simulink model "VehCtrlMdel240926_2018b"  (R2019b)
settings: Solver=FixedStepDiscrete  StartTime=0.0  StopTime=10.0  FixedStep=0.0005  RelTol=1e-3  EnableMultiTasking=on
values from neighbouring files (symbols this model uses):
  Ax_OffSet = 0.0    [VehCtrlMdelDictionary.sldd]
  Ay_OffSet = 0.0    [VehCtrlMdelDictionary.sldd]
  Caf = 460.0    [VehCtrlMdelDictionary.sldd]    (also in trqvparameter.m = 460)
  Car = 440.0    [VehCtrlMdelDictionary.sldd]    (also in trqvparameter.m = 440)
  dwf = 1.2    [VehCtrlMdelDictionary.sldd]    (also in trqvparameter.m)
  dwr = 1.2    [VehCtrlMdelDictionary.sldd]    (also in trqvparameter.m)
  h = 0.29    [VehCtrlMdelDictionary.sldd]    (also in trqvparameter.m)
  i1 = 11.4    [VehCtrlMdelDictionary.sldd]    (also in trqvparameter.m)
  i2 = 3.4    [VehCtrlMdelDictionary.sldd]    (also in trqvparameter.m)
  Iz = 105.0    [VehCtrlMdelDictionary.sldd]    (also in trqvparameter.m = 105)
  Kc = 1.0    [VehCtrlMdelDictionary.sldd]    (also in trqvparameter.m = 10)
  Ki = 1.0    [VehCtrlMdelDictionary.sldd]    (also in trqvparameter.m = 20)
  Kp = 2.0    [VehCtrlMdelDictionary.sldd]    (also in trqvparameter.m = 30)
  Ldwf = 1.2    [VehCtrlMdelDictionary.sldd]    (also in trqvparameter.m)
  Ldwr = 1.16    [VehCtrlMdelDictionary.sldd]    (also in trqvparameter.m)
  lf = 0.761    [VehCtrlMdelDictionary.sldd]    (also in trqvparameter.m)
  lr = 0.831    [VehCtrlMdelDictionary.sldd]    (also in trqvparameter.m)
  m = 340.0    [VehCtrlMdelDictionary.sldd]    (also in trqvparameter.m = 340)
  Offset_Angle = 0.0    [VehCtrlMdelDictionary.sldd]
  Qa = 0.1    [VehCtrlMdelDictionary.sldd]    (also in trqvparameter.m)
  Ra = 2.0    [VehCtrlMdelDictionary.sldd]    (also in trqvparameter.m = 2)
  Rt = 0.2    [VehCtrlMdelDictionary.sldd]    (also in trqvparameter.m)
  thr1 = 2.0    [VehCtrlMdelDictionary.sldd]    (also in trqvparameter.m = 2)
  thr2 = 0.5    [VehCtrlMdelDictionary.sldd]    (also in trqvparameter.m)
  thr3 = 0.8    [VehCtrlMdelDictionary.sldd]    (also in trqvparameter.m)
  thr4 = 0.5    [VehCtrlMdelDictionary.sldd]    (also in trqvparameter.m)
  thr5 = -0.5    [VehCtrlMdelDictionary.sldd]    (also in trqvparameter.m)
  TrqRquRate = 0.1    [VehCtrlMdelDictionary.sldd]    (also in trqvparameter.m)
  YawRate_OffSet = 0.0    [VehCtrlMdelDictionary.sldd]
undefined symbols (not defined in the file or in its folder): DiscIntNeverNeededParam, I_AN06_5V, I_AN07_5V, I_AN08_5V, I_AN09_5V, I_SW01_L, I_SW03_L, O_SW12_HS1A, O_SW14_HS1A, PWM3
libraries: simulink x150, ec5744lib x118, canmsglib x18
(part 2 of 6)

== system VehCtrlMdel240926_2018b/OUTPUT/VCU2AMKMCUFL ==
  MCFL_TargetTorque : Inport
  In2 : Inport  Port=2
  function : TriggerPort  TriggerType=function-call  VariantControl=(inherit)
  Bus Selector : BusSelector  OutputSignals=MCFL_TorqueOn,MCFL_DCOn_setpoints,MCFL_DCEnable,errorReset,MCFL_InverterOn
  CAN Pack1 : canmsglib/CAN Pack  CANdbFile=C:\Users\12045\Desktop\DBC\DRe20_dbc_v1.16\DRe20_dbc_v1.16_CAN2.dbc  MsgList=MCFL_SetPoints  MsgName=MCFL_SetPoints  MsgIDType=Standard (11-bit identifier)  MsgIdentifier=386  MsgLength=8  Remote=off  ApplyMinMax=off  BusOutput=off  SignalInfo={'MCFL_TargetTorque','16','16','LE','signed','Standard','0','0.0098','0','-Inf','Inf';'MCFL_TorqueLimitN','48','16','LE','signed','Standard','0','0.0098','0','-Inf','Inf';'MCFL_TorqueLimitP','32','16','LE','signed','Standard','0','0.0098','0','-Inf','Inf';'MCFL_cDCOn','9','1','LE','unsigned','Standard','0','1','0','0','1';'MCFL_cEnable','10','1','LE','unsigned','Standard','0','1','0','0','1';'MCFL_cErrorReset','11','1','LE','unsigned','Standard','0','1','0','0','1';'MCFL_cInverterOn','8','1','LE','unsigned','Standard','0','1','0','0','1';'MCFL_cReserve1','0','8','LE','unsigned','Standard','0','1','0','-Inf','Inf';'MCFL_cReserve2','12','4','LE','unsigned','Standard','0','1','0','-Inf','Inf'}
      settings: SourceProductName=Vehicle Network Toolbox  SourceProductBaseCode=VN  DataFormat=CANdb specified signals
  CANPackMessage : ec5744lib/RapidECU_U3/04CANCommunication/CANPackMessage  datalength=8  sampletime=-1
      settings: SourceProductName=ECUCoder for MPC5744
  CANTransmit : ec5744lib/RapidECU_U3/04CANCommunication/CANTransmit  canmodule=1  canbuffer=8  canmessageid=386  canmessagetype=Standard(11-bit ID)  datalength=8  sampletime=-1
      settings: SourceProductName=ECUCoder for MPC5744
  Constant1 : Constant  Value=0
  Constant2 : Constant  Value=10
  Ground1 : Ground
  Ground2 : Ground
  Switch : Switch  Criteria=u2 ~= 0
  Terminator3 : Terminator
  wires:
  CANPackMessage/1 -> CANTransmit/1
  CAN Pack1/1 -> CANPackMessage/1
  CANTransmit/1 -> Terminator3/1
  MCFL_TargetTorque/1 -> CAN Pack1/1  "MCFL_TargetTorque"
  Constant1/1 -> CAN Pack1/2, Switch/3  "MCFL_TorqueLimitN"
  Bus Selector/2 -> CAN Pack1/4  "<MCFL_DCOn_setpoints>"
  Switch/1 -> CAN Pack1/3  "MCFL_TorqueLimitP"
  Ground1/1 -> CAN Pack1/8  "MCFL_cReserve1"
  Bus Selector/5 -> CAN Pack1/7  "<MCFL_InverterOn>"
  Bus Selector/3 -> CAN Pack1/5  "<MCFL_DCEnable>"
  Ground2/1 -> CAN Pack1/9  "MCFL_cReserve2"
  In2/1 -> Bus Selector/1
  Bus Selector/4 -> CAN Pack1/6  "<errorReset>"
  Bus Selector/1 -> Switch/2  "<MCFL_TorqueOn>"
  Constant2/1 -> Switch/1  "MCFL_TorqueLimitP"

== system VehCtrlMdel240926_2018b/OUTPUT/VCU2AMKMCUFR ==
  <BUS> : Inport
  In1 : Inport  Port=2
  function : TriggerPort  TriggerType=function-call  VariantControl=(inherit)
  Bus Selector : BusSelector  OutputSignals=MCFR_TorqueOn,MCFL_DCOn_setpoints,MCFL_DCEnable,errorReset,MCFL_InverterOn
  CAN Pack1 : canmsglib/CAN Pack  CANdbFile=C:\Users\12045\Desktop\DBC\DRe20_dbc_v1.16\DRe20_dbc_v1.16_CAN2.dbc  MsgList=MCFR_SetPoints  MsgName=MCFR_SetPoints  MsgIDType=Standard (11-bit identifier)  MsgIdentifier=387  MsgLength=8  Remote=off  ApplyMinMax=off  BusOutput=off  SignalInfo={'MCFR_TargetTorque','16','16','LE','signed','Standard','0','0.0098','0','-Inf','Inf';'MCFR_TorqueLimitN','48','16','LE','signed','Standard','0','0.0098','0','-Inf','Inf';'MCFR_TorqueLimitP','32','16','LE','signed','Standard','0','0.0098','0','-Inf','Inf';'MCFR_cDCOn','9','1','LE','unsigned','Standard','0','1','0','0','1';'MCFR_cEnable','10','1','LE','unsigned','Standard','0','1','0','0','1';'MCFR_cErrorReset','11','1','LE','unsigned','Standard','0','1','0','0','1';'MCFR_cInverterOn','8','1','LE','unsigned','Standard','0','1','0','0','1';'MCFR_cReserve1','0','8','LE','unsigned','Standard','0','1','0','-Inf','Inf';'MCFR_cReserve2','12','4','LE','unsigned','Standard','0','1','0','-Inf','Inf'}
      settings: SourceProductName=Vehicle Network Toolbox  SourceProductBaseCode=VN  DataFormat=CANdb specified signals
  CANPackMessage : ec5744lib/RapidECU_U3/04CANCommunication/CANPackMessage  datalength=8  sampletime=-1
      settings: SourceProductName=ECUCoder for MPC5744
  CANTransmit : ec5744lib/RapidECU_U3/04CANCommunication/CANTransmit  canmodule=1  canbuffer=9  canmessageid=387  canmessagetype=Standard(11-bit ID)  datalength=8  sampletime=-1
      settings: SourceProductName=ECUCoder for MPC5744
  Constant : Constant  Value=0
  Constant1 : Constant  Value=10
  Ground : Ground
  Ground1 : Ground
  Switch : Switch  Criteria=u2 ~= 0
  Terminator3 : Terminator
  wires:
  Ground1/1 -> CAN Pack1/9  "MCFR_cReserve2"
  Bus Selector/3 -> CAN Pack1/5  "<MCFL_DCEnable>"
  Bus Selector/4 -> CAN Pack1/6  "<errorReset>"
  Bus Selector/5 -> CAN Pack1/7  "<MCFL_InverterOn>"
  Ground/1 -> CAN Pack1/8  "MCFR_cReserve1"
  Switch/1 -> CAN Pack1/3  "MCFR_TorqueLimitP"
  Bus Selector/2 -> CAN Pack1/4  "<MCFL_DCOn_setpoints>"
  Constant/1 -> CAN Pack1/2, Switch/3  "MCFR_TorqueLimitN"
  CANTransmit/1 -> Terminator3/1
  CAN Pack1/1 -> CANPackMessage/1
  CANPackMessage/1 -> CANTransmit/1
  In1/1 -> CAN Pack1/1
  <BUS>/1 -> Bus Selector/1
  Constant1/1 -> Switch/1  "MCFR_TorqueLimitP"
  Bus Selector/1 -> Switch/2  "<MCFR_TorqueOn>"

== system VehCtrlMdel240926_2018b/OUTPUT/VCU2CLUSTER ==
  In1 : Inport
  TCS : Inport  Port=2
  function : TriggerPort  TriggerType=function-call  VariantControl=Variant
  Bus Selector : BusSelector  OutputSignals=signal2.APPBrk_BUS.Brk_F,signal2.MCU.MCU_state.Trq,signal2.APPBrk_BUS.Acc_POS,signal2.MCU.MCU_pwr.motor_temp,signal2.VehSpd_FLkph,signal2.MCU.MCU_state.Spd_R_kph,signal2.APPBrk_BUS.Brk_R,signal2.MCU.MCU_state.RPM
  Bus Selector1 : BusSelector  OutputSignals=TCS_TrqRequestFinal_Nm,TCS_flgActv
  CAN Pack : canmsglib/CAN Pack  CANdbFile=E:\candbc\cluster.dbc  MsgList=(none)  MsgName=New_Message_1  MsgIDType=Standard (11-bit identifier)  MsgIdentifier=291  MsgLength=8  Remote=off  ApplyMinMax=off  BusOutput=off  SignalInfo={'Brk_F','56','8','LE','signed','Standard','0','30','100','-3740','3910';'TCS_Trq_cmd','40','8','LE','unsigned','Standard','0','1','0','0','255';'TCS_flag','32','8','LE','signed','Standard','0','1','0','-Inf','Inf';'Trq_feedback','48','8','LE','signed','Standard','0','1','0','-128','250';'acc','24','8','LE','unsigned','Standard','0','1','0','0','100';'motor_temp','0','8','LE','unsigned','Standard','0','1','0','0','100';'veh_spd_F','8','8','LE','unsigned','Standard','0','1','0','0','120';'veh_spd_R','16','8','LE','unsigned','Standard','0','1','0','0','120'}
      settings: SourceProductName=Vehicle Network Toolbox  SourceProductBaseCode=VN  DataFormat=CANdb specified signals
  CAN Pack1 : canmsglib/CAN Pack  CANdbFile=E:\candbc\cluster.dbc  MsgList=(none)  MsgName=New_Message_2  MsgIDType=Standard (11-bit identifier)  MsgIdentifier=292  MsgLength=2  Remote=off  ApplyMinMax=off  BusOutput=off  SignalInfo={'Brk_R','0','8','LE','signed','Standard','0','30','100','-Inf','Inf';'RPM_feedback','8','8','LE','signed','Standard','0','1','0','-Inf','Inf'}
      settings: SourceProductName=Simulink Real-Time  SourceProductBaseCode=XP  DataFormat=CANdb specified signals
  CANPackMessage : ec5744lib/RapidECU_U3/04CANCommunication/CANPackMessage  datalength=8  sampletime=-1
      settings: SourceProductName=ECUCoder for MPC5744
  CANPackMessage1 : ec5744lib/HYFCU001/04CANCommunication/CANPackMessage  datalength=8  sampletime=-1
      settings: SourceProductName=ECUCoder for MPC5744
  CANTransmit : ec5744lib/RapidECU_U3/04CANCommunication/CANTransmit  canmodule=0  canbuffer=9  canmessageid=291  canmessagetype=Standard(11-bit ID)  datalength=8  sampletime=-1
      settings: SourceProductName=ECUCoder for MPC5744
  CANTransmit1 : ec5744lib/RapidECU_U3/04CANCommunication/CANTransmit  canmodule=0  canbuffer=10  canmessageid=292  canmessagetype=Standard(11-bit ID)  datalength=8  sampletime=-1
      settings: SourceProductName=ECUCoder for MPC5744
  Terminator1 : Terminator
  Terminator3 : Terminator
  wires:
  CANTransmit/1 -> Terminator3/1
  CANPackMessage/1 -> CANTransmit/1
  CAN Pack/1 -> CANPackMessage/1
  In1/1 -> Bus Selector/1
  Bus Selector/5 -> CAN Pack/7  "<VehSpd_FLkph>"
  Bus Selector/4 -> CAN Pack/6  "<motor_temp>"
  Bus Selector/3 -> CAN Pack/5  "<Acc_POS>"
  Bus Selector/6 -> CAN Pack/8  "<Spd_R_kph>"
  Bus Selector/1 -> CAN Pack/1  "<Brk_F>"
  Bus Selector/2 -> CAN Pack/4  "<Trq>"
  TCS/1 -> Bus Selector1/1
  Bus Selector1/2 -> CAN Pack/3  "<TCS_flgActv>"
  Bus Selector1/1 -> CAN Pack/2  "<TCS_TrqRequestFinal_Nm>"
  Bus Selector/7 -> CAN Pack1/1  "<Brk_R>"
  Bus Selector/8 -> CAN Pack1/2  "<RPM>"
  CAN Pack1/1 -> CANPackMessage1/1
  CANPackMessage1/1 -> CANTransmit1/1
  CANTransmit1/1 -> Terminator1/1

== system VehCtrlMdel240926_2018b/OUTPUT/VCU2EmraxMCU ==
  note: 0: 0Nm
      | 2: Trq mode
  note: 0: N
      | 2:D
  note: 加ramp
  note: 1.spd改成motor_rpm
      | 2.APP_bad改成acc_error
      | 3.设置模式的优先级
      | 4.车轮低负载（悬空），加最高车速限制
  In1 : Inport
  function : TriggerPort  TriggerType=function-call  VariantControl=(inherit)
  Bus Selector : BusSelector  OutputSignals=Trq_CUT,TrqR_cmd,VCU_SpdCmd_Emrax
  CAN Pack1 : canmsglib/CAN Pack  CANdbFile=E:\candbc\MCU_No1.dbc  MsgList=(none)  MsgName=VCU2MCU1_ID1  MsgIDType=Extended (29-bit identifier)  MsgIdentifier=146927393  MsgLength=8  Remote=off  ApplyMinMax=off  BusOutput=off  SignalInfo={'VCU2MCU_Control_mode_ID1','32','8','LE','unsigned','Standard','0','1','0','0','255';'VCU2MCU_Gear_ID1','40','2','LE','unsigned','Standard','0','1','0','0','3';'VCU2MCU_Speed_Limit_ID1','0','16','LE','unsigned','Standard','0','5.000000e-01','-10000','-10000','10000';'VCU2MCU_Torque_Control_ID1','16','16','LE','unsigned','Standard','0','1','0','0','1000'}
      settings: SourceProductName=Vehicle Network Toolbox  SourceProductBaseCode=VN  DataFormat=CANdb specified signals
  CANPackMessage : ec5744lib/RapidECU_U3/04CANCommunication/CANPackMessage  datalength=8  sampletime=-1
      settings: SourceProductName=ECUCoder for MPC5744
  CANTransmit : ec5744lib/RapidECU_U3/04CANCommunication/CANTransmit  canmodule=0  canbuffer=8  canmessageid=146927393  canmessagetype=Extended(29-bit ID)  datalength=8  sampletime=-1
      settings: SourceProductName=ECUCoder for MPC5744
  Cast To Boolean4 : DataTypeConversion  OutDataTypeStr=uint16
  Cast To Boolean6 : DataTypeConversion  OutDataTypeStr=uint16
  Constant13 : Constant  Value=2
  Constant17 : Constant  Value=0
  Constant19 : Constant  Value=2
  Constant20 : Constant  Value=0
  Data Type Conversion1 : DataTypeConversion  OutDataTypeStr=single
  Data Type Conversion2 : DataTypeConversion  OutDataTypeStr=int32
  MeaModule1 : ec5744lib/HYFCU001/07Calibration/MeaModule  signal=Gear_Trs
      settings: SourceProductName=ECUCoder for MPC5744
  MeaModule2 : ec5744lib/HYFCU001/07Calibration/MeaModule  signal=Mode_Trs
      settings: SourceProductName=ECUCoder for MPC5744
  Ramp : simulink/Sources/Ramp  Commented=on  slope=1  start=0  InitialOutput=0
  Switch2 : Switch  Criteria=u2 > Threshold
  Switch3 : Switch  Criteria=u2 > Threshold
  Terminator3 : Terminator
  wires:
  CANTransmit/1 -> Terminator3/1
  CAN Pack1/1 -> CANPackMessage/1
  CANPackMessage/1 -> CANTransmit/1
  MeaModule1/1 -> Cast To Boolean4/1
  Bus Selector/2 -> Data Type Conversion1/1  "<TrqR_cmd>"
  Constant20/1 -> Switch2/1
  Bus Selector/1 -> Switch2/2, Switch3/2  "<Trq_CUT>"
  Constant19/1 -> Switch2/3
  Constant13/1 -> Switch3/3
  Constant17/1 -> Switch3/1
  Switch3/1 -> MeaModule2/1
  Switch2/1 -> MeaModule1/1
  MeaModule2/1 -> Cast To Boolean6/1
  Data Type Conversion1/1 -> CAN Pack1/3
  Data Type Conversion2/1 -> CAN Pack1/4
  Cast To Boolean4/1 -> CAN Pack1/1
  Cast To Boolean6/1 -> CAN Pack1/2
  Bus Selector/3 -> Data Type Conversion2/1  "<VCU_SpdCmd_Emrax>"
  In1/1 -> Bus Selector/1

== system VehCtrlMdel240926_2018b/OUTPUT/WP_OUTPUT ==
  note: 数据类型转换
  aWaterPumpON : Inport
  LoadOfbWaterPump : Inport  Port=2
  function : TriggerPort  TriggerType=function-call  VariantControl=(inherit)
  Cast To Single : DataTypeConversion  OutDataTypeStr=boolean
  Cast To Single1 : DataTypeConversion  OutDataTypeStr=uint16
  Constant : Constant  Value=uint16(1000)  OutDataTypeStr=uint16  SampleTime=-1
  PowerDriverPWM : ec5744lib/RapidECU_U3/03PowerDriverPWM/PowerDriverPWM  channel=114:O_SW12_HS1A/PWM3  sampletime=-1
      settings: SourceProductName=ECUCoder for MPC5744
  PowerDriverSwitch(HS) : ec5744lib/RapidECU_U3/02PowerDriverSwitch/PowerDriverSwitch(HS)  channel=114:O_SW12_HS1A  sampletime=-1
      settings: SourceProductName=ECUCoder for MPC5744
  wires:
  LoadOfbWaterPump/1 -> Cast To Single1/1
  Constant/1 -> PowerDriverPWM/1
  aWaterPumpON/1 -> Cast To Single/1
  Cast To Single/1 -> PowerDriverSwitch(HS)/1
  Cast To Single1/1 -> PowerDriverPWM/2

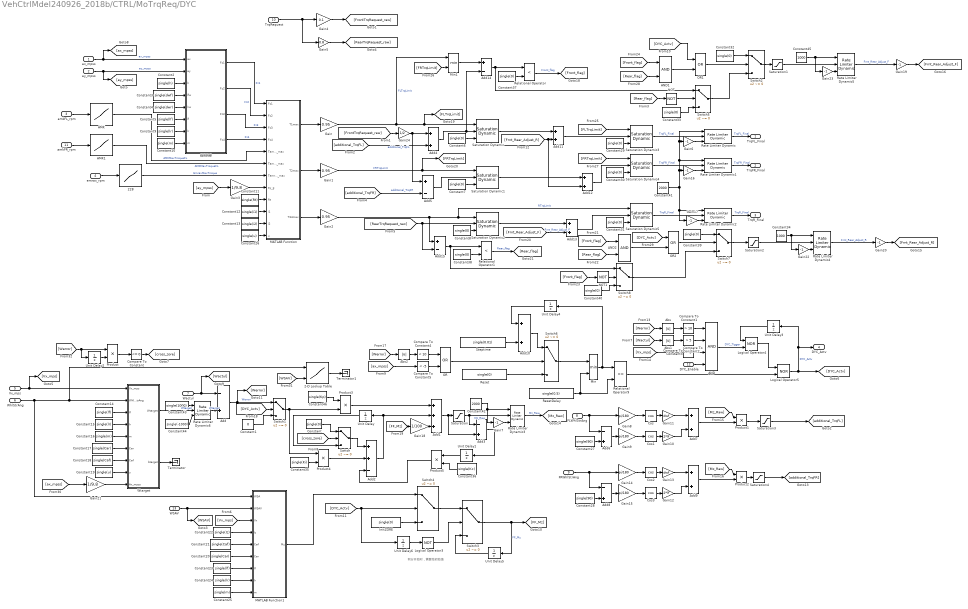
== system VehCtrlMdel240926_2018b/CTRL/MoTrqReq/DYC ==
  note: 积分开始时，需要给初始值
  ax_mpss : Inport
  ay_mpss : Inport  Port=2
  amkFL_rpm : Inport  Port=3
  emrax_rpm : Inport  Port=4
  Vx_mps : Inport  Port=5
  WhlStrAng : Inport  Port=6
  Wactul : Inport  Port=7
  FLWhlStrAng : Inport  Port=8
  FRWhlStrAng : Inport  Port=9
  TrqRequest : Inport  Port=10
  amkFR_rpm : Inport  Port=11
  DYC_Enable : Inport  Port=12
  WSAV : Inport  Port=13
  2-D Lookup Table : Lookup_n-D  BreakpointsForDimension1=[0 5 20 25]  BreakpointsForDimension2=[20 40 60]  Table=[3 5 8;5 8 10;6 10 13;8 12 14]  InternalRulePriority=Speed  RndMeth=Simplest  InputSameDT=on
  228 : Lookup_n-D  NumberOfTableDimensions=1  BreakpointsForDimension1=[200;400;600;800;1000;1200;1400;1600;1800;2000;2200;2400;2600;2800;3000;3200;3400;3600;3800;4000;4200;4400;4600;4800;5000;5200;5400]  BreakpointsForDimension2=[1:3]  Table=[229.85;229.85;229.85;229.85;229.85;229.85;229.85;229.85;229.85;229.85;229.85;229.85;229.46;229.16;228.86;228.86;228.86;228.86;228.86;227.86;227.86;226.87;225.86;224.86;220.86;218.87;215.87]  InternalRulePriority=Speed  RndMeth=Simplest  InputSameDT=on
  AMK : Lookup_n-D  NumberOfTableDimensions=1  BreakpointsForDimension1=[0;1000;2000;3000;4000;5000;6000;7000;8000;9000;10000;11000;12000;13000;14000;15000;16000;17000;18000;19000]  BreakpointsForDimension2=[1:3]  Table=[21;21;21;21;21;21;21;21;21;21;21;21;21;21;20;17.5;15;12.5;8;0]  InternalRulePriority=Speed  RndMeth=Simplest  InputSameDT=on
  AMK1 : Lookup_n-D  NumberOfTableDimensions=1  BreakpointsForDimension1=[0;1000;2000;3000;4000;5000;6000;7000;8000;9000;10000;11000;12000;13000;14000;15000;16000;17000;18000;19000]  BreakpointsForDimension2=[1:3]  Table=[21;21;21;21;21;21;21;21;21;21;21;21;21;21;20;17.5;15;12.5;8;0]  InternalRulePriority=Speed  RndMeth=Simplest  InputSameDT=on
  AND : Logic  Inputs=4  AllPortsSameDT=off  OutDataTypeStr=boolean
  AND1 : Logic  AllPortsSameDT=off  OutDataTypeStr=boolean
  AND2 : Logic  AllPortsSameDT=off  OutDataTypeStr=boolean
  Abs : Abs
  Abs1 : Abs
  Abs2 : Abs
  Add{,3,6,8} (4 alike) : Sum  Inputs=-+
  Add1 : Sum  Inputs=+++
  Add{4,7,9..13} (7 alike) : Sum
  Add14 : Sum  Inputs=+-
  Add15 : Sum  Inputs=+-
  Add2 : Sum  Inputs=++-
  Add5 : Sum  Inputs=+-
  Compare To Constant : simulink/Logic and Bit Operations/Compare To Constant  relop=<=  const=0  OutDataTypeStr=boolean
  Compare To Constant1 : simulink/Logic and Bit Operations/Compare To Constant  relop=>  const=10  OutDataTypeStr=boolean
  Compare To Constant2 : simulink/Logic and Bit Operations/Compare To Constant  relop=>  const=5  OutDataTypeStr=boolean
  Compare To Constant3 : simulink/Logic and Bit Operations/Compare To Constant  relop=>  const=3  OutDataTypeStr=boolean
  Compare To Constant4 : simulink/Logic and Bit Operations/Compare To Constant  relop=<  const=10  OutDataTypeStr=boolean
  Compare To Constant5 : simulink/Logic and Bit Operations/Compare To Constant  relop=<  const=-5  OutDataTypeStr=boolean
  Constant{,6..8,29..33,37..40} (13 alike) : Constant  Value=single(0)
  Constant1 : Constant  Value=0
  Constant10 : Constant  Value=single(m)
  Constant11 : Constant  Value=single(Rt)
  Constant12 : Constant  Value=single(i1)
  Constant13 : Constant  Value=single(i2)
  Constant14 : Constant  Value=single(lf)
  Constant15 : Constant  Value=single(lr)
  Constant16 : Constant  Value=single(m)
  Constant17 : Constant  Value=single(Car)
  Constant18 : Constant  Value=single(Caf)
  Constant19 : Constant  Value=single(u)
  Constant2 : Constant  Value=single(h)
  Constant20 : Constant  Value=single(Car)
  Constant21 : Constant  Value=single(Caf)
  Constant22 : Constant  Value=single(Iz)
  Constant23 : Constant  Value=single(lf)
  Constant24 : Constant  Value=single(lr)
  Constant25 : Constant  Value=single(m)
  Constant26 : Constant  Value=single(u)
  Constant27 : Constant  Value=single(90)
  Constant28 : Constant  Value=single(90)
  Constant3 : Constant  Value=single(dwf)
  Constant34 : Constant  Value=1000
  Constant35 : Constant  Value=single(Ki)
  Constant36 : Constant  Value=single(Kc)
  Constant4 : Constant  Value=single(dwr)
  Constant41 : Constant  Value=2000
  Constant42 : Constant  Value=2000
  Constant43 : Constant  Value=single(1000)
  Constant44 : Constant  Value=single(-1000)
  Constant45 : Constant  Value=1000
  Constant46 : Constant  Value=single(Kp)
  Constant5 : Constant  Value=single(lf)
  Constant9 : Constant  Value=single(lr)
  Cos{,1..3} (4 alike) : Trigonometry  Operator=cos
  Gain : Gain  Gain=0.95
  Gain1 : Gain  Gain=0.95
  Gain10 : Gain  Gain=2*lf
  Gain11 : Gain  Gain=dwf
  Gain12 : Gain  Gain=2*lf
  Gain13 : Gain  Gain=dwf
  Gain{8..9,14..15} (4 alike) : Gain  Gain=pi/180
  Gain{6..7,16..17,19..20,22..23} (8 alike) : Gain  Gain=-1
  Gain18 : Gain  Gain=1/100
  Gain2 : Gain  Gain=0.95
  Gain21 : Gain  Gain=1/9.8
  Gain24 : Gain  Gain=1/2
  Gain3 : Gain  Gain=1/9.8
  Gain4 : Gain  Gain=0.1
  Gain5 : Gain  Gain=0.8
  InitZORE : Constant  Value=single(0)
  Logical Operator3 : Logic  Operator=NOT  AllPortsSameDT=off  OutDataTypeStr=boolean
  Logical Operator4 : Logic  Operator=NOR  AllPortsSameDT=off  OutDataTypeStr=boolean
  Logical Operator5 : Logic  Operator=NOR  AllPortsSameDT=off  OutDataTypeStr=boolean
  MATLAB Function : MATLAB Function  TreatAsAtomicUnit=on
  MATLAB Function1 : MATLAB Function  TreatAsAtomicUnit=on
  Min : MinMax  Inputs=2
  Min1 : MinMax  Inputs=2
  NOT : Logic  Operator=NOT  AllPortsSameDT=off  OutDataTypeStr=boolean
  NOT1 : Logic  Operator=NOT  AllPortsSameDT=off  OutDataTypeStr=boolean
  OR : Logic  Operator=OR  AllPortsSameDT=off  OutDataTypeStr=boolean
  OR1 : Logic  Operator=OR  AllPortsSameDT=off  OutDataTypeStr=boolean
  OR2 : Logic  Operator=OR  AllPortsSameDT=off  OutDataTypeStr=boolean
  Product{,1..5} (6 alike) : Product
  Rate Limiter Dynamic{,1..6} (7 alike) : simulink/Discontinuities/Rate Limiter Dynamic
      settings: SourceProductName=Simulink
  Relational Operator : RelationalOperator  Operator=<  OutDataTypeStr=boolean  RndMeth=Simplest
  Relational Operator1 : RelationalOperator  Operator=<  OutDataTypeStr=boolean  RndMeth=Simplest
  Relational Operator9 : RelationalOperator  OutDataTypeStr=boolean  RndMeth=Simplest
  Reset : Constant  Value=single(0)
  ResetDelay : Constant  Value=single(0.5)
  Saturation : Saturate  UpperLimit=1000  LowerLimit=-1000
  Saturation Dynamic{,1..5} (6 alike) : simulink/Discontinuities/Saturation Dynamic  OutMin=[]  OutMax=[]  OutDataTypeStr=Inherit: Same as second input  OutDataType=fixdt(1, 16)  OutScaling=2^-10  DoSatur=off
  Saturation1 : Saturate  UpperLimit=100  LowerLimit=0
  Saturation2 : Saturate  UpperLimit=100  LowerLimit=0
  Saturation3 : Saturate  UpperLimit=20  LowerLimit=-20
  Saturation4 : Saturate  UpperLimit=20  LowerLimit=-20
  Steptime : Constant  Value=single(0.01)
  Switch{,1..8} (9 alike) : Switch  Criteria=u2 ~= 0
  Terminator : Terminator
  Terminator1 : Terminator
  Unit Delay{,1..6} (7 alike) : UnitDelay  SampleTime=-1  HasFrameUpgradeWarning=on
  Wtarget : MATLAB Function  TreatAsAtomicUnit=on
  载荷转移 : MATLAB Function  TreatAsAtomicUnit=on
  TrqFL_Final : Outport
  TrqFR_Final : Outport  Port=2
  TrqR_Final : Outport  Port=3
  DYC_Actv : Outport  Port=4
  wires:
  Gain5/1 -> [RearTrqRequest_raw]
  [WSAV] -> 2-D Lookup Table/2
  Constant38/1 -> Relational Operator1/2
  Saturation Dynamic5/1 -> Rate Limiter Dynamic2/2  "TrqR_Final"
  MATLAB Function1/1(Mz) -> Switch4/1
  [additional_TrqFL] -> Add4/2  "additional_TrqFL"
  Constant42/1 -> Rate Limiter Dynamic3/1, Gain7/1
  AMK1/1 -> MATLAB Function/6(TamkFR_max)  "AMKMaxTroqueFL"
  Gain15/1 -> Cos3/1
  Gain3/1 -> MATLAB Function/8(ay_g)
  载荷转移/3(Fz3) -> MATLAB Function/3(Fz3)  "Fz3"
  Rate Limiter Dynamic3/1 -> [Mz_Raw]  "Mz_Raw"
  AND1/1 -> OR1/2
  Constant3/1 -> 载荷转移/4(lfw)
  Gain17/1 -> Rate Limiter Dynamic2/3
  Constant35/1 -> Product4/2
  Gain19/1 -> [Frnt_Rear_Adjust_F]
  Gain20/1 -> [Frnt_Rear_Adjust_R]
  [ax_mpss] -> Gain21/1
  [Rear_flag] -> AND1/2
  [cross_zore] -> Switch/2
  [DYC_Actv] -> Switch1/2
  Gain21/1 -> Wtarget/9(Ax_mpss)
  Constant41/1 -> Rate Limiter Dynamic/1, Gain6/1, Rate Limiter Dynamic1/1, Gain16/1, Gain17/1, Rate Limiter Dynamic2/1
  Constant25/1 -> MATLAB Function1/9(m)
  Constant14/1 -> Wtarget/3(lf)
  Gain8/1 -> Cos/1
  NOT1/1 -> Switch8/2
  Saturation/1 -> Rate Limiter Dynamic3/2, Add3/1  "Mz_Raw"
  amkFR_rpm/1 -> AMK1/1
  Gain6/1 -> Rate Limiter Dynamic/3
  [FrontTrqRequest_raw] -> Gain24/1
  [FF_Mz] -> Gain18/1
  [Front_flag] -> AND2/1
  [Mz_Raw] -> Product2/1
  Saturation Dynamic3/1 -> Rate Limiter Dynamic/2  "TrqFL_Final"
  Compare To Constant3/1 -> AND/3
  Rate Limiter Dynamic1/1 -> TrqFR_Final/1  "TrqFR_Final"
  Constant20/1 -> MATLAB Function1/6(Car)
  Rate Limiter Dynamic/1 -> TrqFL_Final/1  "TrqFL_Final"
  Constant16/1 -> Wtarget/5(m)
  Constant9/1 -> 载荷转移/7(lr)
  Constant15/1 -> Wtarget/4(lr)
  Switch6/1 -> Min/1
  [Rear_flag] -> AND2/2
  [RearTrqRequest_raw] -> Saturation Dynamic2/2, Add15/2
  MATLAB Function/3(T34max) -> Gain2/1
  Gain4/1 -> [FrontTrqRequest_raw]
  Product4/1 -> Add2/2
  Product3/1 -> Add1/1
  [Vx_mps] -> MATLAB Function1/3(Vx)
  Constant/1 -> Switch/1
  Constant10/1 -> 载荷转移/8(m)
  [Mz_Raw] -> Product1/1
  Constant2/1 -> 载荷转移/3(h)
  Constant17/1 -> Wtarget/6(Car)
  Constant5/1 -> 载荷转移/6(lf)
  载荷转移/1(Fz1) -> MATLAB Function/1(Fz1)  "Fz1"
  Wactul/1 -> Add/1, [Wactul]
  Switch/1 -> Add2/1
  [Rear_flag] -> NOT/1
  [Werror] -> Abs2/1
  Constant21/1 -> MATLAB Function1/5(Caf)
  Add4/1 -> Add14/2, Saturation Dynamic/2
  Constant26/1 -> MATLAB Function/12(u)
  AMK/1 -> MATLAB Function/5(TamkFL_max)  "AMKMaxTroqueFL"
  Constant12/1 -> MATLAB Function/10(i1)
  [Front_flag] -> NOT1/1
  Constant8/1 -> Saturation Dynamic2/3
  Constant27/1 -> Add6/2
  FRWhlStrAng/1 -> Gain14/1, Add8/1
  ay_mpss/1 -> 载荷转移/2(ay), [ay_mpss]  "ay_mpss"
  AND2/1 -> OR2/2
  Constant22/1 -> MATLAB Function1/4(Iz)
  Unit Delay1/1 -> Product5/1
  Constant4/1 -> 载荷转移/5(lrw)
  Cos1/1 -> Gain10/1
  Gain11/1 -> Add7/1
  Constant36/1 -> Product5/2
  Add2/1 -> Add1/2, Unit Delay/1
  Add13/1 -> Saturation Dynamic5/2
  Constant19/1 -> Wtarget/8(u)
  Constant23/1 -> MATLAB Function1/7(lf)
  Constant18/1 -> Wtarget/7(Caf)
  载荷转移/2(Fz2) -> MATLAB Function/2(Fz2)  "Fz2"
  [DYC_Actv] -> OR2/1
  Gain10/1 -> Add7/2
  Relational Operator9/1 -> Logical Operator5/2
  Switch4/1 -> Switch3/1
  [Front_flag] -> AND1/1
  Constant13/1 -> MATLAB Function/11(i2)
  Saturation Dynamic/1 -> Add11/1
  Add1/1 -> Saturation/1, Add3/2
  Compare To Constant2/1 -> AND/2
  OR1/1 -> Switch2/2
  Switch8/1 -> Switch7/3
  Constant33/1 -> Switch5/3
  ax_mpss/1 -> [ax_mpss], 载荷转移/1(ax)  "ax_mpss"
  Min1/1 -> Add14/1
  Constant40/1 -> Switch8/3
  载荷转移/4(Fz4) -> MATLAB Function/4(Fz4)  "Fz4"
  [ay_mpss] -> Gain3/1
  Reset/1 -> Switch6/3
  Constant24/1 -> MATLAB Function1/8(lr)
  Logical Operator5/1 -> [DYC_Actv], Unit Delay3/1, DYC_Actv/1  "DYC_Actv"
  Constant37/1 -> Relational Operator/2
  [DYC_Actv] -> OR1/1
  Switch5/1 -> Switch2/3
  Saturation Dynamic4/1 -> Rate Limiter Dynamic1/2  "TrqFR_Final"
  Wtarget/2(btarget) -> Terminator/1
  2-D Lookup Table/1 -> Terminator1/1
  [Wactul] -> Abs1/1
  Gain9/1 -> Cos1/1
  Add14/1 -> Relational Operator/1, Switch5/1
  Constant32/1 -> Switch2/1
  228/1 -> MATLAB Function/7(Temrax_max)  "EmraxMaxTroque"
  emrax_rpm/1 -> 228/1
  Constant7/1 -> Saturation Dynamic1/3
  Relational Operator1/1 -> [Rear_flag]  "Rear_flag"
  Constant29/1 -> Saturation Dynamic3/3
  Product5/1 -> Add2/3
  [Frnt_Rear_Adjust_R] -> Add12/2, Add11/2
  MATLAB Function/2(T2max) -> Gain1/1
  [FLTrqLimit] -> Saturation Dynamic3/1
  Compare To Constant4/1 -> OR/1
  FLWhlStrAng/1 -> Add6/1, Gain8/1
  Add6/1 -> Gain9/1
  Unit Delay4/1 -> Add10/1
  Constant11/1 -> MATLAB Function/9(Rt)
  Saturation Dynamic2/1 -> Add13/1
  [DYC_Actv] -> Unit Delay6/1, Switch4/2
  Logical Operator4/1 -> Logical Operator5/1
  Unit Delay3/1 -> Logical Operator4/1
  Constant31/1 -> Saturation Dynamic5/3
  Abs2/1 -> Compare To Constant4/1
  Compare To Constant1/1 -> AND/1
  TrqRequest/1 -> Gain5/1, Gain4/1
  Vx_mps/1 -> Wtarget/1(Vx_mps), [Vx_mps]
  [FRTrqLimit] -> Min1/2
  ResetDelay/1 -> Relational Operator9/2, Min/2
  [ax_mpss] -> Compare To Constant5/1
  Add15/1 -> Switch8/1, Relational Operator1/1
  amkFL_rpm/1 -> AMK/1
  Relational Operator/1 -> [Front_flag]  "Front_flag"
  Unit Delay2/1 -> Product/2
  Constant1/1 -> Switch1/3
  [FRTrqLimit] -> Saturation Dynamic4/1
  Product2/1 -> Saturation4/1
  Switch1/1 -> Product4/1, Product3/2
  Abs1/1 -> Compare To Constant2/1
  Abs/1 -> Compare To Constant1/1
  OR/1 -> Switch6/2
  Constant6/1 -> Saturation Dynamic/3
  Add5/1 -> Saturation Dynamic1/2
  WhlStrAng/1 -> Wtarget/2(WhlStrAng), 2-D Lookup Table/1, MATLAB Function1/1(WSA)
  Product1/1 -> Saturation3/1
  InitZORE/1 -> Switch4/3
  Rate Limiter Dynamic6/1 -> Add/2  "Wtarget"
  Add3/1 -> Unit Delay1/1
  Gain2/1 -> Add15/1, Saturation Dynamic5/1, Saturation Dynamic2/1  "RTrqLimit"
  Unit Delay/1 -> Switch/3
  NOT/1 -> Switch5/2
  Gain13/1 -> Add9/1
  Gain14/1 -> Cos2/1
  OR2/1 -> Switch7/2
  Min/1 -> Unit Delay4/1, Relational Operator9/1
  Add9/1 -> Product2/2
  Compare To Constant5/1 -> OR/2
  Steptime/1 -> Add10/2
  Add/1 -> [Werror], Switch1/1  "Werror"
  Gain1/1 -> [FRTrqLimit], Saturation Dynamic1/1  "FRTrqLimit"
  [additional_TrqFR] -> Add5/2  "additional_TrqFR"
  Constant30/1 -> Saturation Dynamic4/3
  Gain7/1 -> Rate Limiter Dynamic3/3
  Cos3/1 -> Gain12/1
  Unit Delay5/1 -> Switch3/3
  Add10/1 -> Switch6/1
  [Werror] -> Abs/1
  Saturation Dynamic1/1 -> Add12/1
  Product/1 -> Compare To Constant/1
  Rate Limiter Dynamic4/1 -> Gain20/1  "Frnt_Rear_Adjust_R"
  Cos2/1 -> Gain13/1
  Switch3/1 -> [FF_Mz], Unit Delay5/1  "FF_Mz"
  Constant39/1 -> Switch7/1
  Add8/1 -> Gain15/1
  Compare To Constant/1 -> [cross_zore]
  Rate Limiter Dynamic2/1 -> TrqR_Final/1  "TrqR_Final"
  Logical Operator3/1 -> Switch3/2
  Unit Delay6/1 -> Logical Operator3/1
  MATLAB Function/1(T1max) -> Gain/1
  Switch2/1 -> Saturation1/1
  Add7/1 -> Product1/2
  Gain12/1 -> Add9/2
  Gain16/1 -> Rate Limiter Dynamic1/3
  Add11/1 -> Saturation Dynamic3/2
  Add12/1 -> Saturation Dynamic4/2
  Gain/1 -> Min1/1, [FLTrqLimit], Saturation Dynamic/1  "FLTrqLimit"
  AND/1 -> Logical Operator4/2  "DYC_Tigger"
  [Vx_mps] -> Compare To Constant3/1
  [Frnt_Rear_Adjust_F] -> Add13/2  "Frnt_Rear_Adjust_F"
  Constant28/1 -> Add8/2
  Gain18/1 -> Add1/3
  Cos/1 -> Gain11/1
  DYC_Enable/1 -> AND/4
  WSAV/1 -> [WSAV], MATLAB Function1/2(WSAV)
  Rate Limiter Dynamic5/1 -> Gain19/1  "Frnt_Rear_Adjust_F"
  Gain23/1 -> Rate Limiter Dynamic5/3
  Constant45/1 -> Rate Limiter Dynamic5/1, Gain23/1
  Saturation1/1 -> Rate Limiter Dynamic5/2
  Constant34/1 -> Gain22/1, Rate Limiter Dynamic4/1
  Gain22/1 -> Rate Limiter Dynamic4/3
  Switch7/1 -> Saturation2/1
  Saturation2/1 -> Rate Limiter Dynamic4/2
  Saturation3/1 -> [additional_TrqFL]
  Saturation4/1 -> [additional_TrqFR]
  Wtarget/1(Wtarget) -> Rate Limiter Dynamic6/2  "Wtarget"
  Constant43/1 -> Rate Limiter Dynamic6/1
  Constant44/1 -> Rate Limiter Dynamic6/3
  [Werror] -> Unit Delay2/1, Product/1
  Constant46/1 -> Product3/1
  Gain24/1 -> Add5/1, Add4/1

== system VehCtrlMdel240926_2018b/CTRL/MoTrqReq/Subsystem ==
  SingleAMKPowerLimit_KW : Inport
  SingleEmraxPowerLimit_KW : Inport  Port=2
  MCFL_ActualVelocity : Inport  Port=3
  MCFR_ActualVelocity : Inport  Port=4
  RPM : Inport  Port=5
  Add : Sum  Inputs=+-
  Add1 : Sum
  Add2 : Sum
  Add3 : Sum
  Add4 : Sum  Inputs=+-
  Constant : Constant
  Constant1 : Constant  Value=single(9550)  OutDataTypeStr=single
  Constant2 : Constant  Value=single(9550)  OutDataTypeStr=single
  Constant3 : Constant
  Constant5 : Constant  Value=single(9550)  OutDataTypeStr=single
  Divide : Product  Inputs=*/
  Divide1 : Product  Inputs=*/
  Divide2 : Product  Inputs=*/
  Max : MinMax  Function=max  Inputs=2
  Max1 : MinMax  Function=max  Inputs=2
  Max2 : MinMax  Function=max  Inputs=2
  MaxPwr : Constant  Value=single(63)  OutDataTypeStr=single
  MaxPwr1 : Constant  Value=single(7)  OutDataTypeStr=single
  MaxPwr2 : Constant  Value=single(7)  OutDataTypeStr=single
  Product{,1..5} (6 alike) : Product
  RPM_min : Constant  Value=single(10)  OutDataTypeStr=single
  RPM_min1 : Constant  Value=single(1)  OutDataTypeStr=single
  RPM_min2 : Constant  Value=single(10)  OutDataTypeStr=single
  RPM_min3 : Constant  Value=single(1)  OutDataTypeStr=single
  RPM_min4 : Constant  Value=single(10)  OutDataTypeStr=single
  RPM_min5 : Constant  Value=single(1)  OutDataTypeStr=single
  TrqLimEmrax_Nm : Outport
  TrqLimFR_Nm : Outport  Port=2
  TrqLimFL_Nm : Outport  Port=3
  wires:
  Max/1 -> Divide/2
  Divide/1 -> TrqLimEmrax_Nm/1  "TrqLim_Nm"
  RPM_min1/1 -> Max/2
  Constant5/1 -> Product/2
  RPM/1 -> Add1/1
  Product/1 -> Divide/1
  RPM_min/1 -> Add1/2
  Add1/1 -> Max/1
  Add2/1 -> Max1/1
  RPM_min2/1 -> Add2/2
  MaxPwr1/1 -> Product4/1
  Product1/1 -> Divide1/1
  MCFR_ActualVelocity/1 -> Add2/1
  Constant1/1 -> Product1/2
  RPM_min3/1 -> Max1/2
  Divide1/1 -> TrqLimFR_Nm/1  "TrqLim_Nm"
  Max1/1 -> Divide1/2
  Max2/1 -> Divide2/2
  Divide2/1 -> TrqLimFL_Nm/1  "TrqLim_Nm"
  RPM_min5/1 -> Max2/2
  Constant2/1 -> Product2/2
  MCFL_ActualVelocity/1 -> Add3/1
  Product2/1 -> Divide2/1
  RPM_min4/1 -> Add3/2
  Add3/1 -> Max2/1
  MaxPwr/1 -> Product5/1
  Add/1 -> Product5/2
  Product5/1 -> Product/1
  Product3/1 -> Product2/1
  Add4/1 -> Product3/2, Product4/2
  Product4/1 -> Product1/1
  Constant/1 -> Add4/1
  MaxPwr2/1 -> Product3/1
  SingleAMKPowerLimit_KW/1 -> Add4/2
  SingleEmraxPowerLimit_KW/1 -> Add/2
  Constant3/1 -> Add/1

== system VehCtrlMdel240926_2018b/CTRL/MoTrqReq/Subsystem1 ==
  TargetSpdFR : Inport
  AcutSpd : Inport  Port=2
  TrqRqtRawFR : Inport  Port=3
  SpeedLimitEnableFR : Inport  Port=4
  AND : Logic  AllPortsSameDT=off  OutDataTypeStr=boolean
  Add : Sum  Inputs=+-
  Add1 : Sum  Inputs=+++
  Add2 : Sum
  Add4 : Sum
  Add6 : Sum  Inputs=+-
  Compare To Constant : simulink/Logic and Bit Operations/Compare To Constant  relop=<  const=0  OutDataTypeStr=boolean
  Constant{1..3,5} (4 alike) : Constant  Value=0
  Gain : Gain  Gain=20
  Gain1 : Gain  Gain=5
  Gain3 : Gain  Gain=0
  Gain4 : Gain  Gain=-1
  NOT : Logic  Operator=NOT  AllPortsSameDT=off  OutDataTypeStr=boolean
  Saturation Dynamic : simulink/Discontinuities/Saturation Dynamic  OutMin=[]  OutMax=[]  OutDataTypeStr=Inherit: Same as second input  OutDataType=fixdt(1, 16)  OutScaling=2^-10  DoSatur=off
  Saturation Dynamic1 : simulink/Discontinuities/Saturation Dynamic  OutMin=[]  OutMax=[]  OutDataTypeStr=Inherit: Same as second input  OutDataType=fixdt(1, 16)  OutScaling=2^-10  DoSatur=off
  Switch : Switch  Criteria=u2 ~= 0
  Switch1 : Switch  Criteria=u2 ~= 0
  Unit Delay : UnitDelay  SampleTime=-1  HasFrameUpgradeWarning=on
  Unit Delay3 : UnitDelay  SampleTime=-1  HasFrameUpgradeWarning=on
  TrqRqtFinalFR : Outport
  wires:
  Gain4/1 -> Saturation Dynamic1/3
  TrqRqtRawFR/1 -> Gain4/1, Saturation Dynamic/2, Add4/1
  Gain3/1 -> Add1/2
  Constant5/1 -> Saturation Dynamic1/1
  Switch/1 -> Gain1/1, Unit Delay3/1, Add6/1, Gain/1
  Constant1/1 -> Switch/3
  Add2/1 -> Unit Delay/1, Add1/3
  Gain1/1 -> Add2/1
  Add1/1 -> Saturation Dynamic1/2
  Unit Delay/1 -> Switch1/3
  TargetSpdFR/1 -> Add/1
  Unit Delay3/1 -> Add6/2
  Constant2/1 -> Switch1/1
  Saturation Dynamic/1 -> TrqRqtFinalFR/1
  Constant3/1 -> Saturation Dynamic/3
  Add4/1 -> Saturation Dynamic/1
  Switch1/1 -> Add2/2
  NOT/1 -> Switch1/2
  Gain/1 -> Add1/1
  Add6/1 -> Gain3/1
  Add/1 -> Switch/1, Compare To Constant/1
  Saturation Dynamic1/1 -> Add4/2
  AND/1 -> Switch/2, NOT/1
  AcutSpd/1 -> Add/2
  Compare To Constant/1 -> AND/1
  SpeedLimitEnableFR/1 -> AND/2

== system VehCtrlMdel240926_2018b/CTRL/MoTrqReq/Subsystem2 ==
  TargetSpdFL : Inport
  AcutSpd : Inport  Port=2
  TrqRqtRawFL : Inport  Port=3
  SpeedLimitEnableFL : Inport  Port=4
  AND : Logic  AllPortsSameDT=off  OutDataTypeStr=boolean
  Add : Sum  Inputs=+-
  Add1 : Sum  Inputs=+++
  Add2 : Sum
  Add4 : Sum
  Add6 : Sum  Inputs=+-
  Compare To Constant : simulink/Logic and Bit Operations/Compare To Constant  relop=<  const=0  OutDataTypeStr=boolean
  Constant{1..3,5} (4 alike) : Constant  Value=0
  Gain : Gain  Gain=20
  Gain1 : Gain  Gain=5
  Gain3 : Gain  Gain=0
  Gain4 : Gain  Gain=-1
  NOT : Logic  Operator=NOT  AllPortsSameDT=off  OutDataTypeStr=boolean
  Saturation Dynamic : simulink/Discontinuities/Saturation Dynamic  OutMin=[]  OutMax=[]  OutDataTypeStr=Inherit: Same as second input  OutDataType=fixdt(1, 16)  OutScaling=2^-10  DoSatur=off
  Saturation Dynamic1 : simulink/Discontinuities/Saturation Dynamic  OutMin=[]  OutMax=[]  OutDataTypeStr=Inherit: Same as second input  OutDataType=fixdt(1, 16)  OutScaling=2^-10  DoSatur=off
  Switch : Switch  Criteria=u2 ~= 0
  Switch1 : Switch  Criteria=u2 ~= 0
  Unit Delay : UnitDelay  SampleTime=-1  HasFrameUpgradeWarning=on
  Unit Delay3 : UnitDelay  SampleTime=-1  HasFrameUpgradeWarning=on
  TrqRqtFinalFL : Outport
  wires:
  SpeedLimitEnableFL/1 -> AND/2
  Compare To Constant/1 -> AND/1
  AcutSpd/1 -> Add/2
  AND/1 -> NOT/1, Switch/2
  Saturation Dynamic1/1 -> Add4/2
  Add/1 -> Compare To Constant/1, Switch/1
  Add6/1 -> Gain3/1
  Gain/1 -> Add1/1
  NOT/1 -> Switch1/2
  Switch1/1 -> Add2/2
  Add4/1 -> Saturation Dynamic/1
  Constant3/1 -> Saturation Dynamic/3
  Saturation Dynamic/1 -> TrqRqtFinalFL/1
  Constant2/1 -> Switch1/1
  Unit Delay3/1 -> Add6/2
  TargetSpdFL/1 -> Add/1
  Unit Delay/1 -> Switch1/3
  Add1/1 -> Saturation Dynamic1/2
  Gain1/1 -> Add2/1
  Add2/1 -> Add1/3, Unit Delay/1
  Constant1/1 -> Switch/3
  Switch/1 -> Gain/1, Add6/1, Unit Delay3/1, Gain1/1
  Constant5/1 -> Saturation Dynamic1/1
  Gain3/1 -> Add1/2
  TrqRqtRawFL/1 -> Add4/1, Saturation Dynamic/2, Gain4/1
  Gain4/1 -> Saturation Dynamic1/3

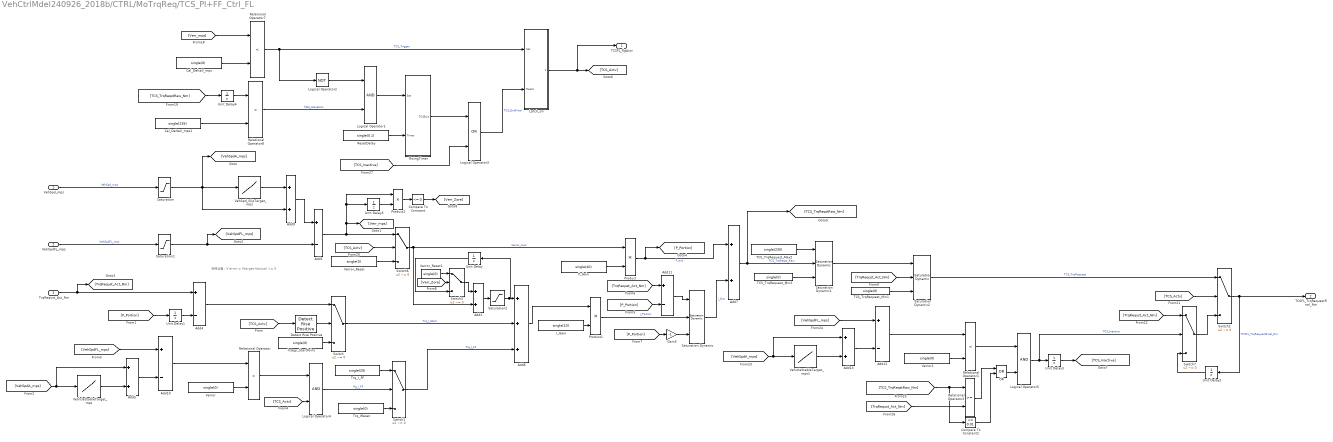
== system VehCtrlMdel240926_2018b/CTRL/MoTrqReq/TCS_PI+FF_Ctrl_FL ==
  note: 特殊设置：V error = Vtarget-Vactual <= 0
  VehSpd_mps : Inport
  VehSpdFL_mps : Inport  Port=2
  TrqRequst_Act_Nm : Inport  Port=3
  Add{1,4,10..12} (5 alike) : Sum  Inputs=+-
  Add{2,5,7,9,13} (5 alike) : Sum
  Add6 : Sum  Inputs=+++
  Cal_DeltaV_mps : Constant  Value=single(0)
  Cal_DeltaV_mps1 : Constant  Value=single(235)
  Compare To Constant : simulink/Logic and Bit Operations/Compare To Constant  relop=<=  const=0  OutDataTypeStr=boolean
  Compare To Constant2 : simulink/Logic and Bit Operations/Compare To Constant  relop=<=  const=0.01  OutDataTypeStr=boolean
  Detect Rise Positive : simulink/Logic and Bit Operations/Detect Rise Positive  vinit=0  OutDataTypeStr=boolean
  Gain3 : Gain  Gain=-1
  I_Gain : Constant  Value=single(10)
  Integr_StartPoint : Constant  Value=single(0)
  Latch_on : Subsystem
  Logical Operator1 : Logic  AllPortsSameDT=off  OutDataTypeStr=boolean
  Logical Operator2 : Logic  Operator=NOT  AllPortsSameDT=off  OutDataTypeStr=boolean
  Logical Operator3 : Logic  Operator=OR  AllPortsSameDT=off  OutDataTypeStr=boolean
  Logical Operator4 : Logic  AllPortsSameDT=off  OutDataTypeStr=boolean
  Logical Operator5 : Logic  AllPortsSameDT=off  OutDataTypeStr=boolean
  OR : Logic  Operator=OR  AllPortsSameDT=off  OutDataTypeStr=boolean
  P_Gain : Constant  Value=single(40)
  Product : Product
  Product1 : Product
  Product2 : Product
  Relational Operator : RelationalOperator  Operator=<  OutDataTypeStr=boolean  RndMeth=Simplest
  Relational Operator1 : RelationalOperator  Operator=<  OutDataTypeStr=boolean  RndMeth=Simplest
  Relational Operator2 : RelationalOperator  OutDataTypeStr=boolean  RndMeth=Simplest
  Relational Operator7 : RelationalOperator  Operator=<  OutDataTypeStr=boolean  RndMeth=Simplest
  Relational Operator8 : RelationalOperator  Operator=>  OutDataTypeStr=boolean  RndMeth=Simplest
  ResetDelay : Constant  Value=single(0.1)
  RisingTimer : Subsystem
  Saturation : Saturate  UpperLimit=40  LowerLimit=0
  Saturation Dynamic : simulink/Discontinuities/Saturation Dynamic  OutMin=[]  OutMax=[]  OutDataTypeStr=Inherit: Same as second input  OutDataType=fixdt(1, 16)  OutScaling=2^-10  DoSatur=off
  Saturation Dynamic1 : simulink/Discontinuities/Saturation Dynamic  OutMin=[]  OutMax=[]  OutDataTypeStr=Inherit: Same as second input  OutDataType=fixdt(1, 16)  OutScaling=2^-10  DoSatur=off
  Saturation Dynamic2 : simulink/Discontinuities/Saturation Dynamic  OutMin=[]  OutMax=[]  OutDataTypeStr=Inherit: Same as second input  OutDataType=fixdt(1, 16)  OutScaling=2^-10  DoSatur=off
  Saturation1 : Saturate  UpperLimit=50  LowerLimit=0
  Saturation2 : Saturate  UpperLimit=400  LowerLimit=-100
  Switch{,1..3,6..7} (6 alike) : Switch  Criteria=u2 ~= 0
  TCS_TrqRequest_Max2 : Constant  Value=single(235)
  TCS_TrqRequest_Min1 : Constant  Value=single(0)
  TCS_TrqRequest_Min2 : Constant  Value=single(0)
  Trq_IReset : Constant  Value=single(0)
  Trq_I_FF : Constant  Value=single(20)
  Unit Delay{,1..5} (6 alike) : UnitDelay  SampleTime=-1  HasFrameUpgradeWarning=on
  VehSpd_SlipTarget_mps : Lookup_n-D  NumberOfTableDimensions=1  BreakpointsForDimension1=[0,3,25,30]  Table=[0.3,0.3,2.5,2.5]  ExtrapMethod=Clip  InternalRulePriority=Speed  RndMeth=Simplest  InputSameDT=on
  VehicleStableTarget_mps : Lookup_n-D  NumberOfTableDimensions=1  BreakpointsForDimension1=[0,3,25,30]  Table=[0.4,0.4,1.2,1.2]  ExtrapMethod=Clip  InternalRulePriority=Speed  RndMeth=Simplest  InputSameDT=on
  VehicleStableTarget_mps1 : Lookup_n-D  NumberOfTableDimensions=1  BreakpointsForDimension1=[0,3,25,30]  Table=[0.4,0.4,1.2,1.2]  ExtrapMethod=Clip  InternalRulePriority=Speed  RndMeth=Simplest  InputSameDT=on
  Verror : Constant  Value=single(0)
  Verror1 : Constant  Value=single(0)
  Verror_Reset : Constant  Value=single(0)
  Verror_Reset1 : Constant  Value=single(0)
  TCSFL_flgActv : Outport
  TCSFL_TrqRequestFinal_Nm : Outport  Port=2
  wires:
  Switch2/1 -> TCSFL_TrqRequestFinal_Nm/1, Unit Delay2/1  "TCSFL_TrqRequestFinal_Nm"
  Saturation/1 -> Add9/2, VehSpd_SlipTarget_mps/1, [VehSpdA_mps]
  Gain3/1 -> Saturation Dynamic/3
  [P_Portion] -> Gain3/1
  P_Gain/1 -> Product/2
  Unit Delay/1 -> Switch3/3
  Add2/1 -> Saturation2/1
  [TrqRequst_Act_Nm] -> Add11/1
  Saturation2/1 -> Unit Delay/1, Add6/1
  Switch/1 -> Add6/2  "Trq_I_Start"
  Saturation Dynamic/1 -> Add7/2  "I_Out"
  VehSpd_mps/1 -> Saturation/1  "VehSpd_mps"
  Saturation1/1 -> Add1/2, [VehSpdFL_mps]
  Product1/1 -> Saturation Dynamic/2  "I_Portion"
  TrqRequst_Act_Nm/1 -> Add4/1, [TrqRequst_Act_Nm]
  Add6/1 -> Product1/1
  TCS_TrqRequest_Min1/1 -> Saturation Dynamic2/3
  Detect Rise Positive/1 -> Switch/2
  Integr_StartPoint/1 -> Switch/3
  I_Gain/1 -> Product1/2
  Saturation Dynamic2/1 -> Switch2/1  "TCS_TrqRequest"
  Add7/1 -> Saturation Dynamic1/2, [TCS_TrqReqstRaw_Nm]  "TCS_TrqReqst_Raw"
  [TrqRequst_Act_Nm] -> Saturation Dynamic2/2
  VehSpd_SlipTarget_mps/1 -> Add9/1
  Add9/1 -> Add1/1
  [Verr_mps] -> Relational Operator7/1
  Cal_DeltaV_mps/1 -> Relational Operator7/2
  Relational Operator7/1 -> Latch_on/1(Set), Logical Operator2/1  "TCS_Trigger"
  [TCS_TrqReqstRaw_Nm] -> Unit Delay4/1
  Logical Operator2/1 -> Logical Operator1/1
  Relational Operator8/1 -> Logical Operator1/2  "fSat_Actuators"
  Cal_DeltaV_mps1/1 -> Relational Operator8/2
  Logical Operator1/1 -> RisingTimer/1(Set)
  ResetDelay/1 -> RisingTimer/2(Timer)
  RisingTimer/1(TCSExit) -> Logical Operator3/1
  Logical Operator3/1 -> Latch_on/2(Reset)  "TCS_ExitFinal"
  Latch_on/1(flg_TCSActv) -> TCSFL_flgActv/1, [TCS_Actv]
  [TCS_Actv] -> Switch6/2
  Verror_Reset/1 -> Switch6/3
  Switch6/1 -> Product/1, Add2/2  "Verror_mps"
  Product/1 -> [P_Portion], Add7/1  "P_out"
  [TCS_Actv] -> Detect Rise Positive/1
  [P_Portion] -> Unit Delay1/1
  Add4/1 -> Switch/1
  Unit Delay1/1 -> Add4/2
  [VehSpdA_mps] -> Add5/1, VehicleStableTarget_mps/1
  VehicleStableTarget_mps/1 -> Add5/2
  Add5/1 -> Add10/2
  [VehSpdFL_mps] -> Add10/1
  Add10/1 -> Relational Operator/1
  Verror/1 -> Relational Operator/2
  Relational Operator/1 -> Logical Operator4/1
  [TCS_Actv] -> Logical Operator4/2
  Logical Operator4/1 -> Switch1/2  "flg_I_FF"
  Trq_I_FF/1 -> Switch1/1
  Trq_IReset/1 -> Switch1/3
  Switch1/1 -> Add6/3  "Trq_I_FF"
  [P_Portion] -> Add11/2
  Add11/1 -> Saturation Dynamic/1
  [TCS_Actv] -> Switch2/2
  Switch7/1 -> Switch2/3
  [TrqRequst_Act_Nm] -> Switch7/1
  Verror1/1 -> Relational Operator1/2
  Add12/1 -> Relational Operator1/1
  [VehSpdFL_mps] -> Add12/1
  Add13/1 -> Add12/2
  VehicleStableTarget_mps1/1 -> Add13/2
  [VehSpdA_mps] -> VehicleStableTarget_mps1/1, Add13/1
  [TCS_TrqReqstRaw_Nm] -> Compare To Constant2/1, Relational Operator2/1
  [TrqRequst_Act_Nm] -> Relational Operator2/2
  Relational Operator1/1 -> Logical Operator5/1
  Logical Operator5/1 -> Switch7/2, Unit Delay3/1  "TCS_Inactive"
  Unit Delay3/1 -> [TCS_Inactive]
  [TCS_Inactive] -> Logical Operator3/2
  Unit Delay4/1 -> Relational Operator8/1
  VehSpdFL_mps/1 -> Saturation1/1  "VehSpdFL_mps"
  Saturation Dynamic1/1 -> Saturation Dynamic2/1
  TCS_TrqRequest_Max2/1 -> Saturation Dynamic1/1
  TCS_TrqRequest_Min2/1 -> Saturation Dynamic1/3
  Switch3/1 -> Add2/1
  Verror_Reset1/1 -> Switch3/1
  [Verr_Zore] -> Switch3/2
  Product2/1 -> Compare To Constant/1
  Unit Delay5/1 -> Product2/2
  Add1/1 -> Switch6/1, [Verr_mps], Unit Delay5/1, Product2/1
  Compare To Constant/1 -> [Verr_Zore]
  Unit Delay2/1 -> Switch7/3
  Compare To Constant2/1 -> OR/2
  Relational Operator2/1 -> OR/1
  OR/1 -> Logical Operator5/2
